simulink model "ball2"  (Simulink 4.00)
settings: Solver=ode45  StartTime=0.0  StopTime=20.0  MaxStep=0.1  RelTol=1e-3
libraries: simulink3 x1
settings Model: LastModifiedBy=Administrator  Refine=3  BlockReductionOpt=off

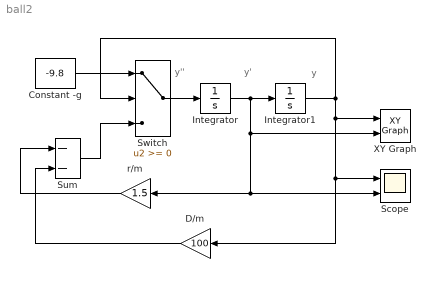
== system ball2 ==
  note: y''
  note: y'
  note: y
  Constant -g : Constant  Value=-9.8
  D/m : Gain  Orientation=left  Gain=100  Multiplication=Element-wise(K.*u)  SaturateOnIntegerOverflow=on
  Integrator : Integrator  ExternalReset=none  InitialConditionSource=internal  InitialCondition=0  LimitOutput=off  UpperSaturationLimit=inf  LowerSaturationLimit=-inf  ShowSaturationPort=off  ShowStatePort=off  AbsoluteTolerance=auto
  Integrator1 : Integrator  ExternalReset=none  InitialConditionSource=internal  InitialCondition=10  LimitOutput=off  UpperSaturationLimit=inf  LowerSaturationLimit=-inf  ShowSaturationPort=off  ShowStatePort=off  AbsoluteTolerance=auto
  Scope : Scope  NumInputPorts=2
      settings: TimeRange=auto  YMin=-5~-5  YMax=5~5  SaveToWorkspace=off  SaveName=ScopeData  LimitDataPoints=on  MaxDataPoints=5000
  Sum : Sum  Inputs=--  SaturateOnIntegerOverflow=on
  Switch : Switch  Threshold=0
  XY Graph : simulink3/Sinks/XY Graph  xmin=-3  xmax=10  ymin=-20  ymax=20  st=0
  r/m : Gain  Orientation=left  Gain=1.5  Multiplication=Element-wise(K.*u)  SaturateOnIntegerOverflow=on
  wires:
  Constant -g/1 -> Switch/1
  Switch/1 -> Integrator/1
  Integrator/1 -> Integrator1/1, r/m/1, Scope/2, XY Graph/2
  Integrator1/1 -> Switch/2, Scope/1, D/m/1, XY Graph/1
  Sum/1 -> Switch/3
  r/m/1 -> Sum/1
  D/m/1 -> Sum/2
